simulink model "new_nncontroller_5_50"  (R2021a)
(part 10 of 14)

  "IW{4,3}(50,:)'" : Constant  Value=[0.033053507094233207375122418625323916785418987274169921875;0.2973426806311201264776400421396829187870025634765625;0.464501186461814985495522023484227247536182403564453125;0.73354913629959395127144716752809472382068634033203125;-0.39041368540470244852258474566042423248291015625;0.062339538682069761676984853693284094333648681640625;0.3923176023164212100624581580632366240024566650390625;0.832229320337579014932316567865200340747833251953125;0.92915156504300089324033251614309847354888916015625;-0.2432649044920278669223989709280431270599365234375;0.84745431286266181825084231604705564677715301513671875;-0.8206999590468477823179682673071511089801788330078125;0.2061179071276242613652840418581035919487476348876953125;-0.0017438841795950695175154709914977502194233238697052001953125;-0.26186691617436841372779099401668645441532135009765625;0.8299568267017625178283424247638322412967681884765625;0.510425409103526295240271792863495647907257080078125;-0.8873622639940652589984892983920872211456298828125;-0.780850934397600671132977367960847914218902587890625;-0.5551955908336381195766762175480835139751434326171875;-0.973847751782330295355905036558397114276885986328125;-0.85763734269972269341764103955938480794429779052734375;0.64362086994668743500369600951671600341796875;0.266624368999497374232987567665986716747283935546875;-0.92486158421116348993251676802174188196659088134765625;-0.5530573542074896931097782726283185184001922607421875;-0.211098839914897862257703309296630322933197021484375;0.84750378509229928880586157902143895626068115234375;-0.093742953628105585295315904659219086170196533203125;-0.3426536774370274596179797299555502831935882568359375;0.70413827402531026233845068418304435908794403076171875;-0.2799052170101139491720232399529777467250823974609375;-0.2867116250029957402745139916078187525272369384765625;-0.5270103929331420022919019174878485500812530517578125;0.5889616478317238890127782724448479712009429931640625;0.99414475823015957534067865708493627607822418212890625;0.82853311201548718312182018053135834634304046630859375;0.497377170580966865287564360187388956546783447265625;-0.197834360036200640475811951546347700059413909912109375;-0.7922772261115884617765914299525320529937744140625;0.50939117083603857594198416336439549922943115234375;0.12013501369103184168718456703572883270680904388427734375;0.2716590404110956757932626715046353638172149658203125;-0.679421651447410734903087359271012246608734130859375;-0.7906125874588898483352750190533697605133056640625;-0.35729324539010642869385492303990758955478668212890625;-0.8900900168257830369356042865547351539134979248046875;-0.8540287367622507730402503511868417263031005859375;0.45002081464119292331105270932312123477458953857421875;-0.8486295752306978190659947358653880655765533447265625]
      mask Display: e = 0.06;c1 = [120 150 230]/255;c2 = ([120 150 230]+0)/383;c3 = ([120 150 230]+128)/383;patch([0 1 1 0],[0 0 1 1],c1);patch([0 1 1 1-e 1-e 0+e],[0 0 1 1-e 0+e 0+e],c2);patch([0 0 1 1-e 0+e 0+e],[0 1 1 1-e 1-e 0+e],c3);plot([0 1 1 0 0],[0 0 1 1 0]);disp('weights');
  "IW{4,3}(6,:)'" : Constant  Value=[0.1886678199041973424954221627558581531047821044921875;0.6723471388729951314644495141692459583282470703125;0.21568666702892702602412100532092154026031494140625;-0.6656034167011257718371552982716821134090423583984375;0.9827314172990997409584679189720191061496734619140625;-0.6244750937782825861432911551673896610736846923828125;0.758497171725523333662977165658958256244659423828125;0.0027318834564258320796170664834789931774139404296875;-0.9777141679848124766749606351368129253387451171875;-0.80436832953686110414537324686534702777862548828125;-0.2883949015228310930325505978544242680072784423828125;-0.6867473337799980814821765306987799704074859619140625;-0.6075214860829787344442820540280081331729888916015625;0.1326230582627285770058733760379254817962646484375;0.36633136361478335629726643674075603485107421875;0.862381952594710288195756220375187695026397705078125;0.7869465778347943807347064648638479411602020263671875;-0.2145935632891478039852017900557257235050201416015625;0.9672621485180836753414723716559819877147674560546875;0.04253748406629398459699586965143680572509765625;-0.194943553000918701201271687750704586505889892578125;0.116591243842754987980470104957930743694305419921875;-0.5169176596321671812717113425605930387973785400390625;-0.845195701062702919870162077131681144237518310546875;0.2176670361043473445050722148152999579906463623046875;-0.7313254385690057812752229438046924769878387451171875;-0.1468774328147552932222197341616265475749969482421875;0.8696648701938780590126043534837663173675537109375;-0.6192324111655793661412872097571380436420440673828125;0.5982523658574192548798009738675318658351898193359375;-0.0629106295557504413551441757590509951114654541015625;0.863873861494384609471808289526961743831634521484375;0.689394475904796077969649559236131608486175537109375;-0.3900873857121001098136048312881030142307281494140625;0.5433504600064329448372291153646074235439300537109375;0.06981630881029499136047888896428048610687255859375;0.16291924806474611386875039897859096527099609375;-0.73629119287367128521282211295329034328460693359375;-0.7051525744130280326515958222444169223308563232421875;0.281949372267346287657119319192133843898773193359375;-0.0844425350039046396233288760413415729999542236328125;0.45442419132731881603604051633737981319427490234375;-0.44632995963872001965455638128332793712615966796875;-0.0018000768572161707226086946320720016956329345703125;0.5350461175271277181053619642625562846660614013671875;0.63746227412696754299759049899876117706298828125;0.06853242156566974330189623287878930568695068359375;0.0932223772568725461695748890633694827556610107421875;-0.5520464640879401141404514419264160096645355224609375;-0.967300176167188663356455435859970748424530029296875]
      mask Display: e = 0.06;c1 = [120 150 230]/255;c2 = ([120 150 230]+0)/383;c3 = ([120 150 230]+128)/383;patch([0 1 1 0],[0 0 1 1],c1);patch([0 1 1 1-e 1-e 0+e],[0 0 1 1-e 0+e 0+e],c2);patch([0 0 1 1-e 0+e 0+e],[0 1 1 1-e 1-e 0+e],c3);plot([0 1 1 0 0],[0 0 1 1 0]);disp('weights');
  "IW{4,3}(7,:)'" : Constant  Value=[-0.266210615213566814674095439841039478778839111328125;-0.81491665986854844305753431399352848529815673828125;-0.3057777733644846396288130563334561884403228759765625;-0.9243628446663632036717217488330788910388946533203125;-0.27477647712149888548083254136145114898681640625;0.4917981813590113215894916720571927726268768310546875;0.4368199508863870317298960799234919250011444091796875;-0.387918334811085951940867744269780814647674560546875;0.592533410150269279625945273437537252902984619140625;0.6243473195949580389907396238413639366626739501953125;0.8802266941767538099838930065743625164031982421875;-0.6860482636179268123299834769568406045436859130859375;0.6096619125959150675697628685156814754009246826171875;0.118168010527158084954635342000983655452728271484375;0.9587896644677049717842010068125091493129730224609375;-0.938899026487839183374717322294600307941436767578125;0.655431162789294585735433429363183677196502685546875;-0.20783252854389377972665897686965763568878173828125;0.375873363734119170231906537082977592945098876953125;0.042903733770204954822702347883023321628570556640625;-0.6610188564177044145964146082405932247638702392578125;0.5301395359915861416055804511415772140026092529296875;-0.1734557892309440685352228683768771588802337646484375;-0.0341349657135487927206440872396342456340789794921875;-0.5927285655708505185401691051083616912364959716796875;-0.524378683695766678596328347339294850826263427734375;0.7063214873819421146805552780278958380222320556640625;-0.9901416367088404779650545606273226439952850341796875;-0.431418669400135623703818055219016969203948974609375;-0.63836892138217304903946569538675248622894287109375;-0.396951507665933345236908280639909207820892333984375;0.964010814654269854173662679386325180530548095703125;0.129295149912215467935538981691934168338775634765625;-0.1368362940825555984503125728224404156208038330078125;-0.4622445756297384189537069687503390014171600341796875;0.79537298662105282431866726255975663661956787109375;-0.450474323930044828756535935099236667156219482421875;-0.78178941950413882722159542026929557323455810546875;0.049903582849598393522683181799948215484619140625;-0.1178137449774776523980790443602018058300018310546875;0.4818494624721356700547403306700289249420166015625;-0.7281174037291939793448136697406880557537078857421875;-0.6041983454394028729694809953798539936542510986328125;-0.7388601071487215232735934478114359080791473388671875;0.137900819599922730418484206893481314182281494140625;0.6189731980105410702464041605708189308643341064453125;0.413269204645541510245720928651280701160430908203125;0.8785741220249148053511589750996790826320648193359375;0.26270874935085775092602489166893064975738525390625;-0.9268197983841413023498034817748703062534332275390625]
      mask Display: e = 0.06;c1 = [120 150 230]/255;c2 = ([120 150 230]+0)/383;c3 = ([120 150 230]+128)/383;patch([0 1 1 0],[0 0 1 1],c1);patch([0 1 1 1-e 1-e 0+e],[0 0 1 1-e 0+e 0+e],c2);patch([0 0 1 1-e 0+e 0+e],[0 1 1 1-e 1-e 0+e],c3);plot([0 1 1 0 0],[0 0 1 1 0]);disp('weights');
  "IW{4,3}(8,:)'" : Constant  Value=[0.459587935049552864796851281425915658473968505859375;0.6184920511126303921400904073379933834075927734375;-0.78074457109660488907110220679896883666515350341796875;0.58042841688706692249155594254261814057826995849609375;-0.436699056139200347814721681061200797557830810546875;-0.68882493689419010962637912598438560962677001953125;-0.0991764743589464980999537146999500691890716552734375;-0.08400239807325569907359152921344502829015254974365234375;-0.7910050324269501942353599588386714458465576171875;0.369241368049827212161062561790458858013153076171875;0.1955332449801164551583809725343598984181880950927734375;-0.5571474177379160952483516666688956320285797119140625;0.06433669599762692481448311809799633920192718505859375;0.149462877157377549419692286392091773450374603271484375;-0.60724627592833224642987488550716079771518707275390625;-0.0125170306166572931072522578688221983611583709716796875;-0.882820693358066233003000888857059180736541748046875;0.313486755433123764902347829774953424930572509765625;0.219731534649916071533226613610167987644672393798828125;-0.774818625087424717179374056286178529262542724609375;-0.040222332792871906548270999337546527385711669921875;-0.1875835559016258979880831248010508716106414794921875;0.3259615557182609091313452154281549155712127685546875;0.2109993719396907330132506785957957617938518524169921875;0.1464145778135289843735478143571526743471622467041015625;-0.3440315498566317575779294202220626175403594970703125;-0.043162583507546210814798115507073816843330860137939453125;-0.83277420795014467369554722608882002532482147216796875;-0.14143824928196446766293092878186143934726715087890625;0.438568743006185091104498496861197054386138916015625;0.64099932052698960216474688422749750316143035888671875;-0.158811620249593499210050140391103923320770263671875;0.60568901381740480882598376410896889865398406982421875;0.3568980729392745576689094377798028290271759033203125;-0.0567595450431124248780179186724126338958740234375;0.5392969375731546666230542541597969830036163330078125;-0.6719667484257261236280101002193987369537353515625;-0.1269190247346221600555082886785385198891162872314453125;0.56291827679822736829606810715631581842899322509765625;-0.44114760087729421034197230255813337862491607666015625;-0.4723798124366067607837749164900742471218109130859375;0.728248049831286881072855976526625454425811767578125;-0.2616863311138943881672958013950847089290618896484375;0.76734357204748915304293177541694603860378265380859375;-0.7150994467998839088096474370104260742664337158203125;0.467737015671206679545690576560446061193943023681640625;-0.83232739879062955790089972651912830770015716552734375;-0.519509320494734083695220761001110076904296875;0.73201155644432513991404221087577752768993377685546875;0.8592193085610642100391487474553287029266357421875]
      mask Display: e = 0.06;c1 = [120 150 230]/255;c2 = ([120 150 230]+0)/383;c3 = ([120 150 230]+128)/383;patch([0 1 1 0],[0 0 1 1],c1);patch([0 1 1 1-e 1-e 0+e],[0 0 1 1-e 0+e 0+e],c2);patch([0 0 1 1-e 0+e 0+e],[0 1 1 1-e 1-e 0+e],c3);plot([0 1 1 0 0],[0 0 1 1 0]);disp('weights');
  "IW{4,3}(9,:)'" : Constant  Value=[0.8414721279922747765311896728235296905040740966796875;-0.4203307339091877370407246417016722261905670166015625;0.7686681455509880578347292612306773662567138671875;0.6081109977899761265263123277691192924976348876953125;0.4443330523268109732981656634365208446979522705078125;-0.845667464993120621130628933315165340900421142578125;0.9623514439113802776404327232739888131618499755859375;-0.6808733459184621583659691168577410280704498291015625;-0.6300650397854681283860145413200370967388153076171875;-0.507755165562193244710442741052247583866119384765625;-0.3263592523376168674786867995862849056720733642578125;-0.261045392509544171844027005136013031005859375;-0.929156376674756590006154510774649679660797119140625;0.1254504270012120059618609957396984100341796875;0.77043584801936848549530623131431639194488525390625;-0.7395947558750834982532751382677815854549407958984375;-0.5955762807238931255682246046490035951137542724609375;-0.974594454715600466698788295616395771503448486328125;0.4462665782316517226746555024874396622180938720703125;0.657633415951217603634404440526850521564483642578125;0.21653665044997172373086868901737034320831298828125;0.77820875660911870141944746137596666812896728515625;0.3535903222427154712903529798495583236217498779296875;-0.1517401425614848253786703935475088655948638916015625;-0.3371601180451395673998149504768662154674530029296875;-0.69776792036756862813717816607095301151275634765625;-0.8407066871415533881872761412523686885833740234375;0.451562154924749048490184577531181275844573974609375;0.4567709085685418557432058150880038738250732421875;-0.6612043229407580380296849398291669785976409912109375;0.998282647979549242478469750494696199893951416015625;-0.1260555097547211289565893821418285369873046875;-0.8594841142688662838367008589557372033596038818359375;-0.3782641162049025229663357094977982342243194580078125;0.8253835893855645533534470814629457890987396240234375;-0.5553725962505406954505815519951283931732177734375;-0.478782767938145337183186711627058684825897216796875;-0.521078144856089497949369615525938570499420166015625;-0.29114256224827528285459266044199466705322265625;0.1742793304007275168032720102928578853607177734375;0.830201953595627539783663451089523732662200927734375;0.606738343784695377536309024435468018054962158203125;0.0179159942370283875590075695072300732135772705078125;0.014290526648512269503044080920517444610595703125;-0.8055936389486506588042402654536999762058258056640625;-0.0009638815375858644785012074862606823444366455078125;0.4386869176296552819138696577283553779125213623046875;0.7961490067084089350402109630522318184375762939453125;0.6091542504429681148536701584816910326480865478515625;0.302153481360535547395329558639787137508392333984375]
      mask Display: e = 0.06;c1 = [120 150 230]/255;c2 = ([120 150 230]+0)/383;c3 = ([120 150 230]+128)/383;patch([0 1 1 0],[0 0 1 1],c1);patch([0 1 1 1-e 1-e 0+e],[0 0 1 1-e 0+e 0+e],c2);patch([0 0 1 1-e 0+e 0+e],[0 1 1 1-e 1-e 0+e],c3);plot([0 1 1 0 0],[0 0 1 1 0]);disp('weights');
  Mux : Mux  Inputs=50
      mask Display: e = 0.06;c1 = [120 150 230]/255;c2 = ([120 150 230]+0)/383;c3 = ([120 150 230]+128)/383;patch([0 1 1 0],[0 0 1 1],c1);patch([0 1 1 1-e 1-e 0+e],[0 0 1 1-e 0+e 0+e],c2);patch([0 0 1 1-e 0+e 0+e],[0 1 1 1-e 1-e 0+e],c3);plot([0 1 1 0 0],[0 0 1 1 0]);disp('Mux');
  dotprod{1..50} (50 alike) : neural/Weight Functions/dotprod
  "lz{4,3}" : Outport
      mask Display: e = 0.06;c1 = [120 230 180]/255;c2 = ([120 230 180]+0)/(256+128);c3 = ([120 230 180]+128)/(256+128);patch([0 1 1 0],[0 0 1 1],c1);patch([0 1 1 1-e 1-e 0+e],[0 0 1 1-e 0+e 0+e],c2);patch([0 0 1 1-e 0+e 0+e],[0 1 1 1-e 1-e 0+e],c3);plot([0 1 1 0 0],[0 0 1 1 0]);
  wires:
  "IW{4,3}(1,:)'"/1 -> dotprod1/1
  "ad{4,3}"/1 -> dotprod1/2, dotprod2/2, dotprod3/2, dotprod4/2, dotprod5/2, dotprod6/2, dotprod7/2, dotprod8/2, dotprod9/2, dotprod10/2, dotprod11/2, dotprod12/2, dotprod13/2, dotprod14/2, dotprod15/2, dotprod16/2, dotprod17/2, dotprod18/2, dotprod19/2, dotprod20/2, dotprod21/2, dotprod22/2, dotprod23/2, dotprod24/2, dotprod25/2, dotprod26/2, dotprod27/2, dotprod28/2, dotprod29/2, dotprod30/2, dotprod31/2, dotprod32/2, dotprod33/2, dotprod34/2, dotprod35/2, dotprod36/2, dotprod37/2, dotprod38/2, dotprod39/2, dotprod40/2, dotprod41/2, dotprod42/2, dotprod43/2, dotprod44/2, dotprod45/2, dotprod46/2, dotprod47/2, dotprod48/2, dotprod49/2, dotprod50/2
  dotprod1/1 -> Mux/1
  "IW{4,3}(2,:)'"/1 -> dotprod2/1
  dotprod2/1 -> Mux/2
  "IW{4,3}(3,:)'"/1 -> dotprod3/1
  dotprod3/1 -> Mux/3
  "IW{4,3}(4,:)'"/1 -> dotprod4/1
  dotprod4/1 -> Mux/4
  "IW{4,3}(5,:)'"/1 -> dotprod5/1
  dotprod5/1 -> Mux/5
  "IW{4,3}(6,:)'"/1 -> dotprod6/1
  dotprod6/1 -> Mux/6
  "IW{4,3}(7,:)'"/1 -> dotprod7/1
  dotprod7/1 -> Mux/7
  "IW{4,3}(8,:)'"/1 -> dotprod8/1
  dotprod8/1 -> Mux/8
  "IW{4,3}(9,:)'"/1 -> dotprod9/1
  dotprod9/1 -> Mux/9
  "IW{4,3}(10,:)'"/1 -> dotprod10/1
  dotprod10/1 -> Mux/10
  "IW{4,3}(11,:)'"/1 -> dotprod11/1
  dotprod11/1 -> Mux/11
  "IW{4,3}(12,:)'"/1 -> dotprod12/1
  dotprod12/1 -> Mux/12
  "IW{4,3}(13,:)'"/1 -> dotprod13/1
  dotprod13/1 -> Mux/13
  "IW{4,3}(14,:)'"/1 -> dotprod14/1
  dotprod14/1 -> Mux/14
  "IW{4,3}(15,:)'"/1 -> dotprod15/1
  dotprod15/1 -> Mux/15
  "IW{4,3}(16,:)'"/1 -> dotprod16/1
  dotprod16/1 -> Mux/16
  "IW{4,3}(17,:)'"/1 -> dotprod17/1
  dotprod17/1 -> Mux/17
  "IW{4,3}(18,:)'"/1 -> dotprod18/1
  dotprod18/1 -> Mux/18
  "IW{4,3}(19,:)'"/1 -> dotprod19/1
  dotprod19/1 -> Mux/19
  "IW{4,3}(20,:)'"/1 -> dotprod20/1
  dotprod20/1 -> Mux/20
  "IW{4,3}(21,:)'"/1 -> dotprod21/1
  dotprod21/1 -> Mux/21
  "IW{4,3}(22,:)'"/1 -> dotprod22/1
  dotprod22/1 -> Mux/22
  "IW{4,3}(23,:)'"/1 -> dotprod23/1
  dotprod23/1 -> Mux/23
  "IW{4,3}(24,:)'"/1 -> dotprod24/1
  dotprod24/1 -> Mux/24
  "IW{4,3}(25,:)'"/1 -> dotprod25/1
  dotprod25/1 -> Mux/25
  "IW{4,3}(26,:)'"/1 -> dotprod26/1
  dotprod26/1 -> Mux/26
  "IW{4,3}(27,:)'"/1 -> dotprod27/1
  dotprod27/1 -> Mux/27
  "IW{4,3}(28,:)'"/1 -> dotprod28/1
  dotprod28/1 -> Mux/28
  "IW{4,3}(29,:)'"/1 -> dotprod29/1
  dotprod29/1 -> Mux/29
  "IW{4,3}(30,:)'"/1 -> dotprod30/1
  dotprod30/1 -> Mux/30
  "IW{4,3}(31,:)'"/1 -> dotprod31/1
  dotprod31/1 -> Mux/31
  "IW{4,3}(32,:)'"/1 -> dotprod32/1
  dotprod32/1 -> Mux/32
  "IW{4,3}(33,:)'"/1 -> dotprod33/1
  dotprod33/1 -> Mux/33
  "IW{4,3}(34,:)'"/1 -> dotprod34/1
  dotprod34/1 -> Mux/34
  "IW{4,3}(35,:)'"/1 -> dotprod35/1
  dotprod35/1 -> Mux/35
  "IW{4,3}(36,:)'"/1 -> dotprod36/1
  dotprod36/1 -> Mux/36
  "IW{4,3}(37,:)'"/1 -> dotprod37/1
  dotprod37/1 -> Mux/37
  "IW{4,3}(38,:)'"/1 -> dotprod38/1
  dotprod38/1 -> Mux/38
  "IW{4,3}(39,:)'"/1 -> dotprod39/1
  dotprod39/1 -> Mux/39
  "IW{4,3}(40,:)'"/1 -> dotprod40/1
  dotprod40/1 -> Mux/40
  "IW{4,3}(41,:)'"/1 -> dotprod41/1
  dotprod41/1 -> Mux/41
  "IW{4,3}(42,:)'"/1 -> dotprod42/1
  dotprod42/1 -> Mux/42
  "IW{4,3}(43,:)'"/1 -> dotprod43/1
  dotprod43/1 -> Mux/43
  "IW{4,3}(44,:)'"/1 -> dotprod44/1
  dotprod44/1 -> Mux/44
  "IW{4,3}(45,:)'"/1 -> dotprod45/1
  dotprod45/1 -> Mux/45
  "IW{4,3}(46,:)'"/1 -> dotprod46/1
  dotprod46/1 -> Mux/46
  "IW{4,3}(47,:)'"/1 -> dotprod47/1
  dotprod47/1 -> Mux/47
  "IW{4,3}(48,:)'"/1 -> dotprod48/1
  dotprod48/1 -> Mux/48
  "IW{4,3}(49,:)'"/1 -> dotprod49/1
  dotprod49/1 -> Mux/49
  "IW{4,3}(50,:)'"/1 -> dotprod50/1
  dotprod50/1 -> Mux/50
  Mux/1 -> "lz{4,3}"/1
